simulink model "test234_FF"  (R2021b)
settings: Solver=ode45  StartTime=0.0  StopTime=200  RelTol=1e-3  EnableMultiTasking=on
values from neighbouring files (symbols this model uses):
  Aaf = A-B(:,2)*k_sae    [Codigo_CVOO.m]
  ad_f = atuadores_f    (= 100)    [Codigo_CVOO.m]
  ad_lower_v = 0    [Codigo_CVOO.m]
  ad_upper_v = 5    [Codigo_CVOO.m]
  atuadores_f = 100    [Codigo_CVOO.m]
  atuadores_t = 40 * 0.001    (= 0.04)    [Codigo_CVOO.m]
  atuadores_vmax = 60 * deg    (= 1.0471975512)    [Codigo_CVOO.m]
  B = [0, Ydr ... (first row only)    [Codigo_CVOO.m]
  C = eye(5)    [Codigo_CVOO.m]
  C_kalman = [0 1 0 0 0 ... (first row only)    [Codigo_CVOO.m]
  D = zeros(5,2)    [Codigo_CVOO.m]
  D_kalman = zeros(4,2)    [Codigo_CVOO.m]
  da0 = 0.58*deg    (= 0.0101229096616)    [Codigo_CVOO.m]
  damax = 30*deg    (= 0.523598775598)    [Codigo_CVOO.m]
  deg = pi/180    (= 0.0174532925199)    [Codigo_CVOO.m]
  dr0 = -0.01*deg    (= -0.000174532925199)    [Codigo_CVOO.m]
  drmax = 30*deg    (= 0.523598775598)    [Codigo_CVOO.m]
  g_gain = g_gain_gyro * (5-0)/(g_upper_v-g_lower_v)    (= 0.00833333333333)    [Codigo_CVOO.m]
  g_lower = -300    [Codigo_CVOO.m]
  g_offset = 5 - g_upper * g_gain    (= 2.5)    [Codigo_CVOO.m]
  g_rms = 4.4    [Codigo_CVOO.m]
  g_upper = 300    [Codigo_CVOO.m]
  gps_f = 5    [Codigo_CVOO.m]
  K_int = [K_lqr(1,6), K_lqr(1,7) ... (first row only)    [Codigo_CVOO.m]
  Kc_control = [K_lqr(1,2), K_lqr(1,3), K_lqr(1,5) ... (first row only)    [Codigo_CVOO.m]
  Ky = [K_lqr(1,1), K_lqr(1,4) ... (first row only)    [Codigo_CVOO.m]
  m_lower = -8 * 10^-4    (= -0.0008)    [Codigo_CVOO.m]
  m_rms = 0.015 * 10^-4    (= 1.5e-06)    [Codigo_CVOO.m]
  m_upper = 8 * 10^-4    (= 0.0008)    [Codigo_CVOO.m]
  mag_lisboa_y = 0.004 * 10^-4    (= 4e-07)    [Codigo_CVOO.m]
  mag_lisboa_z = 0.356 * 10^-4    (= 3.56e-05)    [Codigo_CVOO.m]
  R_est = diag([10^(-5) (g_rms)^2 (a_rms)^2 (m_rms)^2])    [Codigo_CVOO.m]
  u0 = 29.2*kn    (= 15.0217777648)    [Codigo_CVOO.m]
undefined symbols (not defined in the file or in its folder): Continuous, Time
libraries: simulink x8, ctrlSharedLib x1
settings Model: Creator=F3SV  LastModifiedBy=Francisco
settings SolverCC: AlgebraicLoopSolver=TrustRegion
settings DataIOCC: LimitDataPoints=on  SaveFormat=Array  SignalLoggingSaveFormat=ModelDataLogs  ReturnWorkspaceOutputs=off
settings OptimizationCC: InitFltsAndDblsToZero=on  LifeSpan=inf
settings DebuggingCC: SaveWithParameterizedLinksMsg=none  UnderspecifiedInitializationDetection=Classic  MergeDetectMultiDrivingBlocksExec=none  SignalResolutionControl=TryResolveAllWithWarning  SolverPrmCheckMsg=warning  MultiTaskDSMMsg=warning  MultiTaskCondExecSysMsg=none  SFUnexpectedBacktrackingDiag=warning  SFNoUnconditionalDefaultTransitionDiag=warning  SFExecutionAtInitializationDiag=none  SFMachineParentedDataDiag=warning  ArithmeticOperatorsInVariantConditions=warning
settings HardwareCC: ProdBitPerPointer=32  ProdBitPerSizeT=32  ProdBitPerPtrDiffT=32  ProdLargestAtomicFloat=None  ProdIntDivRoundTo=Undefined  ProdEndianess=Unspecified  ProdWordSize=32  ProdHWDeviceType=32-bit Generic
settings ModelReferenceCC: PropagateSignalLabelsOutOfModel=off
settings CodeAppCC: StateflowObjectComments=on
settings GRTTargetCC: TargetFcnLib=ansi_tfl_tmw.mat  TargetLangStandard=C89/C90 (ANSI)  CombineOutputUpdateFcns=off  GRTInterface=on
settings ConfigComp: CovMetricSettings=dw  CovSaveCumulativeToWorkspaceVar=on  CovSaveSingleToWorkspaceVar=on

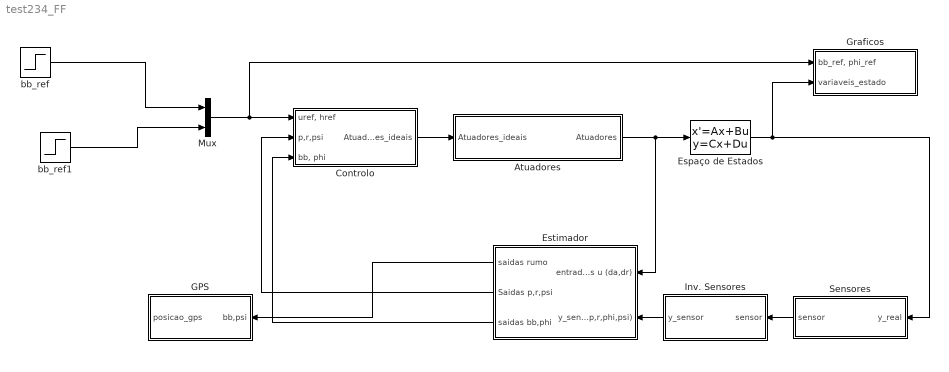
== system test234_FF ==
  Atuadores : Subsystem
  Controlo : Subsystem
  Espaço de Estados : StateSpace  A=Aaf  B=B  C=C  D=D  InitialCondition=[0,0,0,0,0]
  Estimador : Subsystem
  GPS : Subsystem
  Graficos : Subsystem
  Inv. Sensores : Subsystem
  Mux : Mux  Inputs=2
  Sensores : Subsystem
  bb_ref : Step  Time=0  After=0  SampleTime=0
  bb_ref1 : Step  Time=0  After=15*deg  SampleTime=0
  wires:
  Atuadores/1(Atuadores) -> Espaço de Estados/1, Estimador/1(entradas u (da,dr))
  Espaço de Estados/1 -> Graficos/2(variaveis_estado), Sensores/1(y_real)
  Estimador/1(saidas rumo) -> GPS/1(bb,psi)
  bb_ref/1 -> Mux/1
  Controlo/1(Atuadores_ideais) -> Atuadores/1(Atuadores_ideais)
  Mux/1 -> Controlo/1("uref, href"), Graficos/1("bb_ref, phi_ref")
  Sensores/1(sensor) -> Inv. Sensores/1(sensor)
  Inv. Sensores/1(y_sensor) -> Estimador/2(y_sensor (p,r,phi,psi))
  Estimador/3(saidas bb,phi) -> Controlo/3("bb, phi")
  Estimador/2(Saidas p,r,psi) -> Controlo/2(p,r,psi)
  bb_ref1/1 -> Mux/2

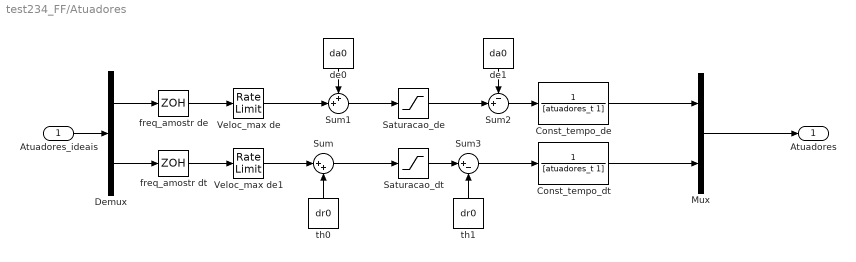
== system test234_FF/Atuadores ==
  Atuadores_ideais : Inport
  Const_tempo_de : TransferFcn  Denominator=[atuadores_t 1]
  "Const_tempo_dt " : TransferFcn  Denominator=[atuadores_t 1]
  Demux : Demux  Outputs=2
  Mux : Mux  Inputs=2
  "Saturacao_de " : Saturate  UpperLimit=damax  LowerLimit=-damax
  Saturacao_dt : Saturate  UpperLimit=drmax  LowerLimit=-drmax
  Sum : Sum  Inputs=|++
  Sum1 : Sum  Inputs=++|
  Sum2 : Sum  Inputs=-+|
  Sum3 : Sum  Inputs=|+-
  Veloc_max de : RateLimiter  RisingSlewLimit=atuadores_vmax  FallingSlewLimit=-atuadores_vmax  SampleTimeMode=inherited
  Veloc_max de1 : RateLimiter  RisingSlewLimit=atuadores_vmax  FallingSlewLimit=-atuadores_vmax  SampleTimeMode=inherited
  de0 : Constant  Value=da0
  de1 : Constant  Value=da0
  freq_amostr de : ZeroOrderHold  SampleTime=1/atuadores_f
  freq_amostr dt : ZeroOrderHold  SampleTime=1/atuadores_f
  th0 : Constant  Value=dr0
  th1 : Constant  Value=dr0
  Atuadores : Outport  VectorParamsAs1DForOutWhenUnconnected=off
  wires:
  Mux/1 -> Atuadores/1
  de1/1 -> Sum2/1
  de0/1 -> Sum1/1
  Saturacao_dt/1 -> Sum3/1
  th0/1 -> Sum/2
  Sum1/1 -> "Saturacao_de "/1
  Sum/1 -> Saturacao_dt/1
  Atuadores_ideais/1 -> Demux/1
  "Saturacao_de "/1 -> Sum2/2
  th1/1 -> Sum3/2
  Demux/2 -> freq_amostr dt/1
  freq_amostr dt/1 -> Veloc_max de1/1
  Demux/1 -> freq_amostr de/1
  Sum2/1 -> Const_tempo_de/1
  freq_amostr de/1 -> Veloc_max de/1
  Veloc_max de/1 -> Sum1/2
  Const_tempo_de/1 -> Mux/1
  Sum3/1 -> "Const_tempo_dt "/1
  "Const_tempo_dt "/1 -> Mux/2
  Veloc_max de1/1 -> Sum/1

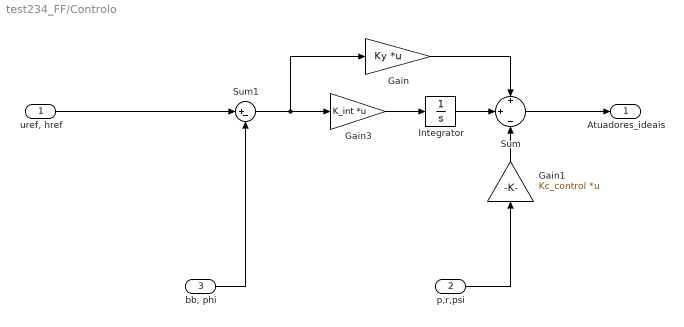
== system test234_FF/Controlo ==
  "uref, href" : Inport
  p,r,psi : Inport  Port=2
  "bb, phi" : Inport  Port=3
  Gain : Gain  Gain=Ky  Multiplication=Matrix(K*u)
  Gain1 : Gain  Gain=Kc_control  Multiplication=Matrix(K*u)
  Gain3 : Gain  Gain=K_int  Multiplication=Matrix(K*u)
  Integrator : Integrator
  Sum : Sum  Inputs=+|+|-
  Sum1 : Sum  Inputs=|+-
  Atuadores_ideais : Outport  VectorParamsAs1DForOutWhenUnconnected=off
  wires:
  Sum1/1 -> Gain3/1, Gain/1
  Gain/1 -> Sum/1
  Integrator/1 -> Sum/2
  Gain1/1 -> Sum/3
  Gain3/1 -> Integrator/1
  "bb, phi"/1 -> Sum1/2
  p,r,psi/1 -> Gain1/1
  Sum/1 -> Atuadores_ideais/1
  "uref, href"/1 -> Sum1/1

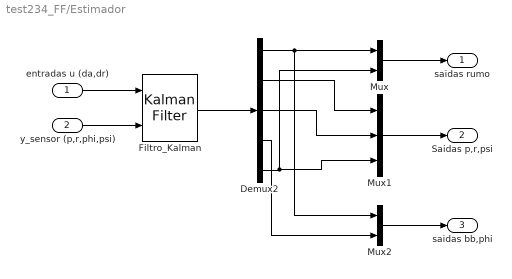
== system test234_FF/Estimador ==
  entradas u (da,dr) : Inport
  y_sensor (p,r,phi,psi) : Inport  Port=2
  Demux2 : Demux  Outputs=5
  Filtro_Kalman : ctrlSharedLib/Kalman Filter  TimeDomain=Continuous-Time  UseCurrentEstimator=on  ModelSource=Individual A, B, C, D matrices  ModelSourceVariable=ss(0.95,1,1,0,1)  A=Aaf  B=B  C=C_kalman  D=D_kalman  NumberOfStates=1  NumberOfInputs=1  NumberOfOutputs=1  InitialEstimateSource=Dialog  X0=[0 0 0 0 0]  P0=10  UseK=off  UseGH=off  NumberOfProcessNoiseInputs=1  G=1  TimeInvariantG=on  H=0  TimeInvariantH=on  Q=Q_est  TimeInvariantQ=on  R=R_est  TimeInvariantR=on  N=0  TimeInvariantN=on  AddInputPort=on  AddEnablePort=off  OutputEstimatedY=off  OutputP=off  Ts=-1
  Mux : Mux  Inputs=2
  Mux1 : Mux  Inputs=3
  Mux2 : Mux  Inputs=2
  saidas rumo : Outport  VectorParamsAs1DForOutWhenUnconnected=off
  Saidas p,r,psi : Outport  Port=2  VectorParamsAs1DForOutWhenUnconnected=off
  saidas bb,phi : Outport  Port=3  VectorParamsAs1DForOutWhenUnconnected=off
  wires:
  Demux2/2 -> Mux1/1
  Mux/1 -> saidas rumo/1
  entradas u (da,dr)/1 -> Filtro_Kalman/1
  Filtro_Kalman/1 -> Demux2/1
  Demux2/1 -> Mux2/1, Mux/1
  Mux1/1 -> Saidas p,r,psi/1
  Demux2/3 -> Mux1/2
  Demux2/5 -> Mux1/3, Mux/2
  y_sensor (p,r,phi,psi)/1 -> Filtro_Kalman/2
  Mux2/1 -> saidas bb,phi/1
  Demux2/4 -> Mux2/2

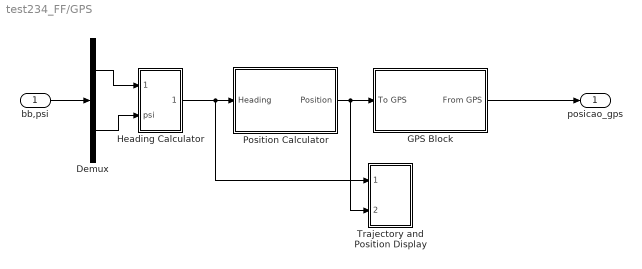
== system test234_FF/GPS ==
  bb,psi : Inport
  Demux : Demux  Outputs=2
  GPS Block : Subsystem
  Heading Calculator : Subsystem
  Position Calculator : Subsystem
  Trajectory and Position Display : Subsystem
  posicao_gps : Outport  VectorParamsAs1DForOutWhenUnconnected=off
  wires:
  Heading Calculator/1(Heading) -> Position Calculator/1(Heading), Trajectory and Position Display/1(Heading)
  Position Calculator/1(Position) -> GPS Block/1(To GPS), Trajectory and Position Display/2(Position)
  Demux/2 -> Heading Calculator/2(psi)
  GPS Block/1(From GPS) -> posicao_gps/1
  bb,psi/1 -> Demux/1
  Demux/1 -> Heading Calculator/1(beta)

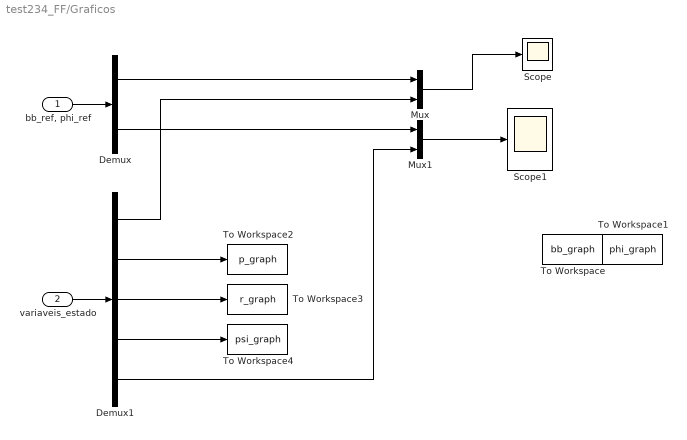
== system test234_FF/Graficos ==
  "bb_ref, phi_ref" : Inport
  variaveis_estado : Inport  Port=2
  Demux : Demux  Outputs=2
  Demux1 : Demux  Outputs=5
  Mux : Mux  Inputs=2
  Mux1 : Mux  Inputs=2
  Scope : Scope
  Scope1 : Scope
  To Workspace : ToWorkspace  VariableName=bb_graph  SaveFormat=Timeseries  SampleTime=-1
  To Workspace1 : ToWorkspace  VariableName=phi_graph  SaveFormat=Timeseries  SampleTime=-1
  To Workspace2 : ToWorkspace  VariableName=p_graph  SaveFormat=Timeseries  SampleTime=-1
  To Workspace3 : ToWorkspace  VariableName=r_graph  SaveFormat=Timeseries  SampleTime=-1
  To Workspace4 : ToWorkspace  VariableName=psi_graph  SaveFormat=Timeseries  SampleTime=-1
  wires:
  "bb_ref, phi_ref"/1 -> Demux/1
  variaveis_estado/1 -> Demux1/1
  Demux/1 -> Mux/1
  Demux1/1 -> Mux/2
  Demux/2 -> Mux1/1
  Demux1/5 -> Mux1/2
  Demux1/2 -> To Workspace2/1
  Demux1/3 -> To Workspace3/1
  Demux1/4 -> To Workspace4/1
  Mux1/1 -> Scope1/1
  Mux/1 -> Scope/1

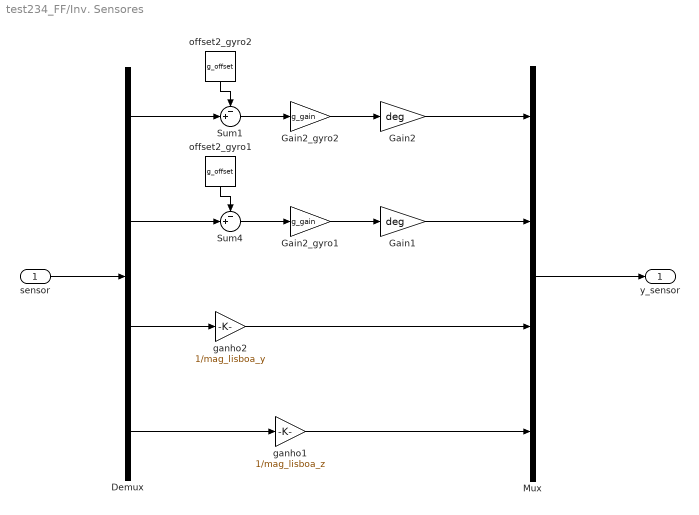
== system test234_FF/Inv. Sensores ==
  sensor : Inport
  Demux : Demux
  Gain1 : Gain  Gain=deg
  Gain2 : Gain  Gain=deg
  Gain2_gyro1 : Gain  Gain=g_gain
  Gain2_gyro2 : Gain  Gain=g_gain
  Mux : Mux
  Sum1 : Sum  Inputs=-+|
  Sum4 : Sum  Inputs=-+|
  ganho1 : Gain  Gain=1/mag_lisboa_z
  ganho2 : Gain  Gain=1/mag_lisboa_y
  offset2_gyro1 : Constant  Value=g_offset
  offset2_gyro2 : Constant  Value=g_offset
  y_sensor : Outport  VectorParamsAs1DForOutWhenUnconnected=off
  wires:
  sensor/1 -> Demux/1
  ganho2/1 -> Mux/3
  Demux/4 -> ganho1/1
  ganho1/1 -> Mux/4
  Demux/3 -> ganho2/1
  Mux/1 -> y_sensor/1
  Demux/2 -> Sum4/2
  Sum4/1 -> Gain2_gyro1/1
  Gain2_gyro1/1 -> Gain1/1
  offset2_gyro1/1 -> Sum4/1
  Gain1/1 -> Mux/2
  Demux/1 -> Sum1/2
  Gain2_gyro2/1 -> Gain2/1
  Gain2/1 -> Mux/1
  offset2_gyro2/1 -> Sum1/1
  Sum1/1 -> Gain2_gyro2/1

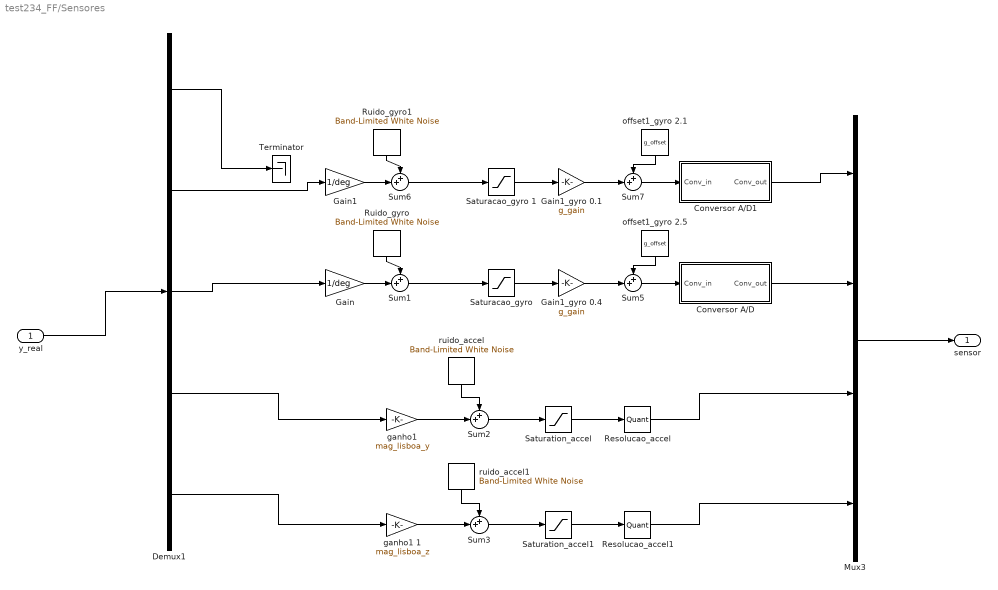
== system test234_FF/Sensores ==
  y_real : Inport
  Conversor A/D : Subsystem
  Conversor A/D1 : Subsystem
  Demux1 : Demux  Outputs=5
  Gain : Gain  Gain=1/deg
  Gain1 : Gain  Gain=1/deg
  Gain1_gyro 0.1 : Gain  Gain=g_gain
  Gain1_gyro 0.4 : Gain  Gain=g_gain
  Mux3 : Mux
  Resolucao_accel : Quantizer  QuantizationInterval=m_res
  Resolucao_accel1 : Quantizer  QuantizationInterval=m_res
  Ruido_gyro : simulink/Sources/Band-Limited White Noise  Cov=(g_rms)^2/atuadores_f  Ts=1/atuadores_f  seed=[745]
  Ruido_gyro1 : simulink/Sources/Band-Limited White Noise  Cov=(g_rms)^2/atuadores_f  Ts=1/atuadores_f  seed=[745]
  "Saturacao_gyro " : Saturate  UpperLimit=g_upper  LowerLimit=g_lower
  Saturacao_gyro 1 : Saturate  UpperLimit=g_upper  LowerLimit=g_lower
  Saturation_accel : Saturate  UpperLimit=m_upper  LowerLimit=m_lower
  Saturation_accel1 : Saturate  UpperLimit=m_upper  LowerLimit=m_lower
  Sum{1..3,5..7} (6 alike) : Sum  Inputs=++|
  Terminator : Terminator
  "ganho1 " : Gain  Gain=mag_lisboa_y
  ganho1 1 : Gain  Gain=mag_lisboa_z
  offset1_gyro 2.1 : Constant  Value=g_offset
  offset1_gyro 2.5 : Constant  Value=g_offset
  ruido_accel : simulink/Sources/Band-Limited White Noise  Cov=(m_rms)^2/atuadores_f  Ts=1/atuadores_f  seed=[37]
  ruido_accel1 : simulink/Sources/Band-Limited White Noise  Cov=(m_rms)^2/atuadores_f  Ts=1/atuadores_f  seed=[37]
  sensor : Outport  VectorParamsAs1DForOutWhenUnconnected=off
  wires:
  y_real/1 -> Demux1/1
  Demux1/1 -> Terminator/1
  Demux1/3 -> Gain/1
  Sum1/1 -> "Saturacao_gyro "/1
  Gain/1 -> Sum1/2
  Ruido_gyro/1 -> Sum1/1
  "ganho1 "/1 -> Sum2/2
  Saturation_accel/1 -> Resolucao_accel/1
  ruido_accel/1 -> Sum2/1
  Resolucao_accel/1 -> Mux3/3
  Demux1/4 -> "ganho1 "/1
  Sum2/1 -> Saturation_accel/1
  Mux3/1 -> sensor/1
  Sum5/1 -> Conversor A/D/1(Conv_in)
  Gain1_gyro 0.4/1 -> Sum5/2
  offset1_gyro 2.5/1 -> Sum5/1
  "Saturacao_gyro "/1 -> Gain1_gyro 0.4/1
  Conversor A/D/1("Conv_out ") -> Mux3/2
  Conversor A/D1/1("Conv_out ") -> Mux3/1
  Saturacao_gyro 1/1 -> Gain1_gyro 0.1/1
  Sum7/1 -> Conversor A/D1/1(Conv_in)
  Gain1/1 -> Sum6/2
  Gain1_gyro 0.1/1 -> Sum7/2
  Ruido_gyro1/1 -> Sum6/1
  Demux1/2 -> Gain1/1
  Sum6/1 -> Saturacao_gyro 1/1
  offset1_gyro 2.1/1 -> Sum7/1
  Demux1/5 -> ganho1 1/1
  Resolucao_accel1/1 -> Mux3/4
  ganho1 1/1 -> Sum3/2
  Saturation_accel1/1 -> Resolucao_accel1/1
  Sum3/1 -> Saturation_accel1/1
  ruido_accel1/1 -> Sum3/1

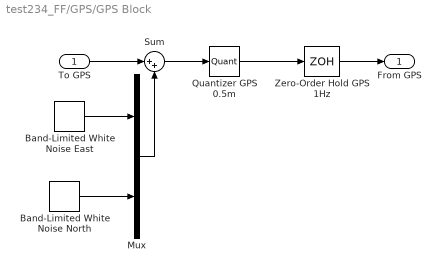
== system test234_FF/GPS/GPS Block ==
  To GPS : Inport
  Band-Limited White Noise East : simulink/Sources/Band-Limited White Noise  Cov=[2^2*0.1]  Ts=0.1  seed=[23341]
  Band-Limited White Noise North : simulink/Sources/Band-Limited White Noise  Cov=[2^2*0.1]  Ts=0.1  seed=[23341]
  Mux : Mux  Inputs=2
  Quantizer GPS 0.5m : Quantizer  QuantizationInterval=gps_p_res
  Sum : Sum  Inputs=|++
  Zero-Order Hold GPS 1Hz : ZeroOrderHold  SampleTime=1/gps_f
  From GPS : Outport
  wires:
  Quantizer GPS 0.5m/1 -> Zero-Order Hold GPS 1Hz/1
  Sum/1 -> Quantizer GPS 0.5m/1
  Mux/1 -> Sum/2
  Band-Limited White Noise East/1 -> Mux/1
  Band-Limited White Noise North/1 -> Mux/2
  Zero-Order Hold GPS 1Hz/1 -> From GPS/1
  To GPS/1 -> Sum/1

== system test234_FF/GPS/Heading Calculator ==
  beta : Inport
  psi : Inport  Port=2
  Sum : Sum  Inputs=|++
  Heading : Outport
  wires:
  Sum/1 -> Heading/1
  beta/1 -> Sum/1
  psi/1 -> Sum/2

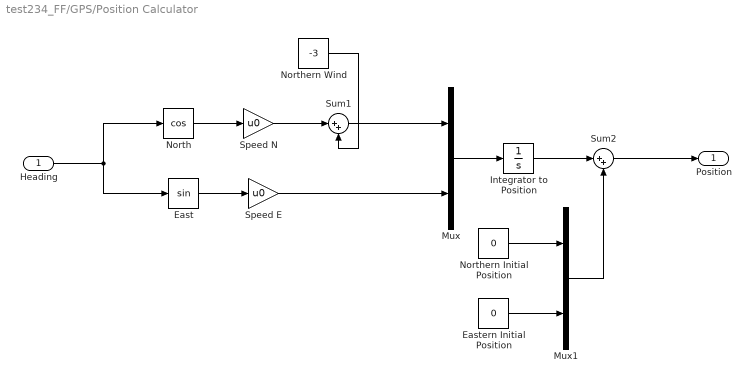
== system test234_FF/GPS/Position Calculator ==
  Heading : Inport
  East : Trigonometry
  Eastern Initial Position : Constant  Value=0
  Integrator to Position : Integrator
  Mux : Mux  Inputs=2
  Mux1 : Mux  Inputs=2
  North : Trigonometry  Operator=cos
  Northern Initial Position : Constant  Value=0
  Northern Wind : Constant  Value=-3
  Speed E : Gain  Gain=u0
  Speed N : Gain  Gain=u0
  Sum1 : Sum  Inputs=|++
  Sum2 : Sum  Inputs=|++
  Position : Outport
  wires:
  North/1 -> Speed N/1
  East/1 -> Speed E/1
  Heading/1 -> East/1, North/1
  Speed N/1 -> Sum1/1
  Sum1/1 -> Mux/1
  Speed E/1 -> Mux/2
  Mux/1 -> Integrator to Position/1
  Integrator to Position/1 -> Sum2/1
  Sum2/1 -> Position/1
  Mux1/1 -> Sum2/2
  Northern Initial Position/1 -> Mux1/1
  Eastern Initial Position/1 -> Mux1/2
  Northern Wind/1 -> Sum1/2

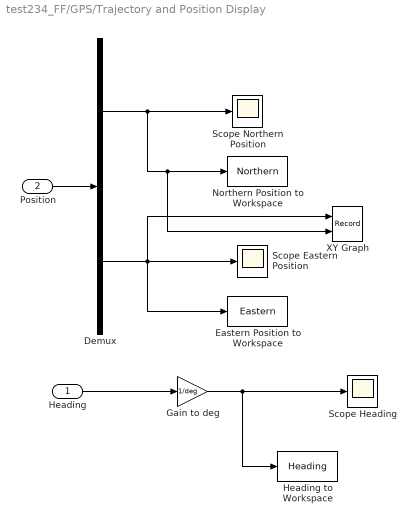
== system test234_FF/GPS/Trajectory and Position Display ==
  Heading : Inport
  Position : Inport  Port=2
  Demux : Demux  Outputs=2
  Eastern Position to Workspace : ToWorkspace  VariableName=Eastern  SampleTime=-1
  Gain to deg : Gain  Gain=1/deg
  Heading to Workspace : ToWorkspace  VariableName=Heading  SaveFormat=Structure  SampleTime=-1
  Northern Position to Workspace : ToWorkspace  VariableName=Northern  SampleTime=-1
  Scope Eastern Position : Scope
  Scope Heading : Scope
  Scope Northern Position : Scope
  XY Graph : Record  FileSettingsInternal="{\"entries\":[{\"content\":{\"excelSettings\":{\"content\":{},\"type\":\"Streamout.ExcelSettings\"}},\"type\":\"Streamout.FileSettingStorage\",\"uuid\":\"7d777ecd-3ca3-45be-b83d-4f9ef6ccb776\"}],\"packageUris\":[\"http://schema.mathworks.com/mf0/streamout_blocks/R2020a\"],\"version\":\"1.0\"}"  Layout=[1 1]  SignalsInternal="{\"entries\":[{\"content\":{\"signals\":[{\"content\":{\"blockPath\":[\"test234/GPS/Trajectory and Position Display/XY Graph\"],\"channel\":[],\"dimensions\":[1],\"domain\":\"test234/GPS/Trajectory and Position Display/XY Graph\",\"lineColor\":\"#a2142f\",\"plots\":[1],\"port\":1,\"sid\":[\"\"],\"signalID\":10345,\"signalName\":\"Demux:2\"},\"type\":\"RecordBlkView.Signal\",\"uuid\":\"333f62d7-6c7c-43aa-93bf-fc14a9954c94\"},{\"content\":{\"blockPath\":[\"test234/GPS/Trajectory and Position Display/XY Graph\"],\"channel\":[],\"dimensions\":[1],\"domain\":\"test234/GPS/Trajectory and Position Display/XY Graph\",\"lineColor\":\"#139fff\",\"plots\":[1],\"port\":2,\"sid\":[\"\"],\"signalID\":10349,\"signalName\":\"Demux:1\"},\"type\":\"RecordBlkView.Signal\",\"uuid\":\"14faffd6-a2d5-4c15-8359-63b6ff4fda1a\"}]},\"type\":\"RecordBlkView.InputSignals\",\"uuid\":\"452e2516-fb76-4abd-a425-8963e6204193\"}],\"packageUris\":[\"http://schema.mathworks.com/mf0/streamout_blocks/R2020a\"],\"version\":\"1.0\"}"  VisualizationBindings="{\"xyplotplugin\":{\"info\":[{\"series\":[{\"bindingParametersList\":[{\"parameter\":\"X-Axis\",\"signalID\":10345,\"signalName\":\"Demux:2\"},{\"parameter\":\"Y-Axis\",\"signalID\":10349,\"signalName\":\"Demux:1\"}],\"seriesID\":10686}],\"subplotID\":1}]}}"  CompatibilityTag=XY  st=-1
  wires:
  Heading/1 -> Gain to deg/1
  Gain to deg/1 -> Scope Heading/1, Heading to Workspace/1
  Demux/1 -> Scope Northern Position/1, Northern Position to Workspace/1, XY Graph/2
  Demux/2 -> Scope Eastern Position/1, Eastern Position to Workspace/1, XY Graph/1
  Position/1 -> Demux/1

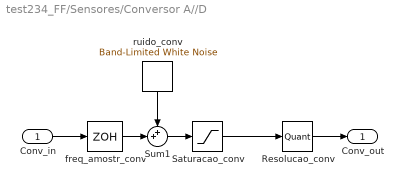
== system test234_FF/Sensores/Conversor A//D ==
  Conv_in : Inport
  "Resolucao_conv " : Quantizer  QuantizationInterval=ad_quantization
  Saturacao_conv : Saturate  UpperLimit=ad_upper_v  LowerLimit=ad_lower_v
  Sum1 : Sum  Inputs=++|
  "freq_amostr_conv " : ZeroOrderHold  SampleTime=1/atuadores_f
  ruido_conv : simulink/Sources/Band-Limited White Noise  Cov=(ad_f)^2/atuadores_f  Ts=1/atuadores_f  seed=[30]
  "Conv_out " : Outport  VectorParamsAs1DForOutWhenUnconnected=off
  wires:
  Conv_in/1 -> "freq_amostr_conv "/1
  "Resolucao_conv "/1 -> "Conv_out "/1
  Sum1/1 -> Saturacao_conv/1
  "freq_amostr_conv "/1 -> Sum1/2
  ruido_conv/1 -> Sum1/1
  Saturacao_conv/1 -> "Resolucao_conv "/1

== system test234_FF/Sensores/Conversor A//D1 ==
  Conv_in : Inport
  "Resolucao_conv " : Quantizer  QuantizationInterval=ad_quantization
  Saturacao_conv : Saturate  UpperLimit=ad_upper_v  LowerLimit=ad_lower_v
  Sum1 : Sum  Inputs=++|
  "freq_amostr_conv " : ZeroOrderHold  SampleTime=1/atuadores_f
  ruido_conv : simulink/Sources/Band-Limited White Noise  Cov=(ad_f)^2/atuadores_f  Ts=1/atuadores_f  seed=[30]
  "Conv_out " : Outport  VectorParamsAs1DForOutWhenUnconnected=off
  wires:
  Conv_in/1 -> "freq_amostr_conv "/1
  "Resolucao_conv "/1 -> "Conv_out "/1
  Sum1/1 -> Saturacao_conv/1
  "freq_amostr_conv "/1 -> Sum1/2
  ruido_conv/1 -> Sum1/1
  Saturacao_conv/1 -> "Resolucao_conv "/1
